simulink model "Rotational_kinematics"  (R2018a)
settings: Solver=VariableStepAuto  StartTime=0.0  StopTime=10  RelTol=1e-3
settings Model: Creator=lamy  LastModifiedBy=lamy

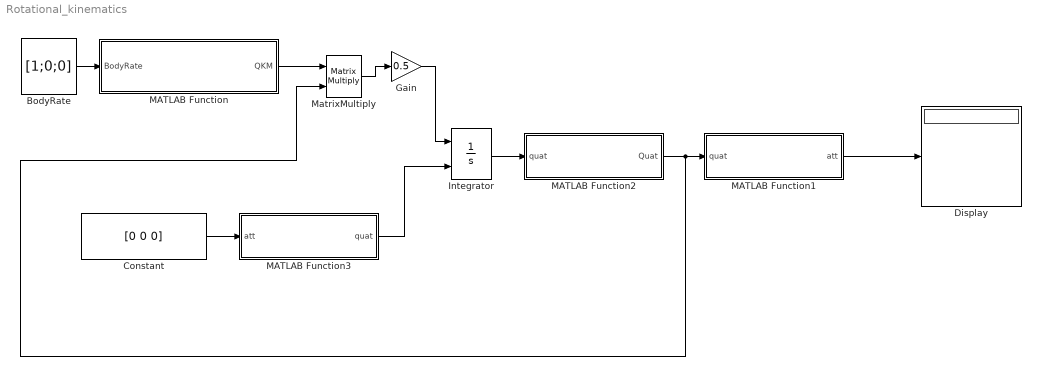
== system Rotational_kinematics ==
  BodyRate : Constant  Value=[1;0;0]  VectorParams1D=off
  Constant : Constant  Value=[0 0 0]
  Display : Display
  Gain : Gain  Gain=0.5
  Integrator : Integrator  InitialConditionSource=external
  MATLAB Function : MATLAB Function  TreatAsAtomicUnit=on
  MATLAB Function1 : MATLAB Function  TreatAsAtomicUnit=on
  MATLAB Function2 : MATLAB Function  TreatAsAtomicUnit=on
  MATLAB Function3 : MATLAB Function  TreatAsAtomicUnit=on
  MatrixMultiply : Product  Multiplication=Matrix(*)
  wires:
  BodyRate/1 -> MATLAB Function/1(BodyRate)
  MATLAB Function1/1(att) -> Display/1
  MATLAB Function3/1(quat) -> Integrator/2
  Constant/1 -> MATLAB Function3/1(att)
  Gain/1 -> Integrator/1
  MATLAB Function/1(QKM) -> MatrixMultiply/1
  MatrixMultiply/1 -> Gain/1
  Integrator/1 -> MATLAB Function2/1(quat)
  MATLAB Function2/1(Quat) -> MatrixMultiply/2, MATLAB Function1/1(quat)

== matlab function Rotational_kinematics/MATLAB Function1 ==
  data: quat input; att output
function att = quat2att(quat)
yaw = atan2(2*(quat(1)*quat(4) + quat(2)*quat(3)), 1-2*(quat(3)^2 + quat(4)^2));
pitch = asin(2*(quat(1)*quat(3) - quat(2)*quat(4)));
roll = atan2(2*(quat(1)*quat(2) + quat(3)*quat(4)), 1-2*(quat(2)^2 + quat(3)^2));
att = [roll; pitch; yaw];

== matlab function Rotational_kinematics/MATLAB Function ==
  data: BodyRate input; QKM output
function QKM = RotKin(BodyRate)
p=BodyRate(1);
q=BodyRate(2);
r=BodyRate(3);
QKM=[ 0,-p,-q,-r;
p, 0, r,-q;
q,-r, 0, p;
r, q,-p, 0];
%q = 0.5*(QKM*quat);

== matlab function Rotational_kinematics/MATLAB Function2 ==
  data: quat input; Quat output
function Quat = quat_normalize(quat)
norm = dot(quat,quat);
Quat = quat/norm;

== matlab function Rotational_kinematics/MATLAB Function3 ==
  data: att input; quat output
function quat = att2quat(att)
quat = [0;0;0;0];
quat(1) = cos(att(1)/2)*cos(att(2)/2)*cos(att(3)/2) + sin(att(1)/2)*sin(att(2)/2)*sin(att(3)/2);
quat(2) = sin(att(1)/2)*cos(att(2)/2)*cos(att(3)/2) - cos(att(1)/2)*sin(att(2)/2)*sin(att(3)/2);
quat(3) = cos(att(1)/2)*sin(att(2)/2)*cos(att(3)/2) + sin(att(1)/2)*cos(att(2)/2)*sin(att(3)/2);
quat(4) = cos(att(1)/2)*cos(att(2)/2)*sin(att(3)/2) - sin(att(1)/2)*sin(att(2)/2)*cos(att(3)/2);
